simulink model "car_model2"  (R2023a)
settings: Solver=ode14x  StartTime=0.0  StopTime=40  FixedStep=0.001  RelTol=1e-3  EnableMultiTasking=on
undefined symbols (not defined in the file or in its folder): DiscIntNeverNeededParam, magnitude
settings Model: Creator=Sıla The Magnificent  LastModifiedBy=Sıla The Magnificent

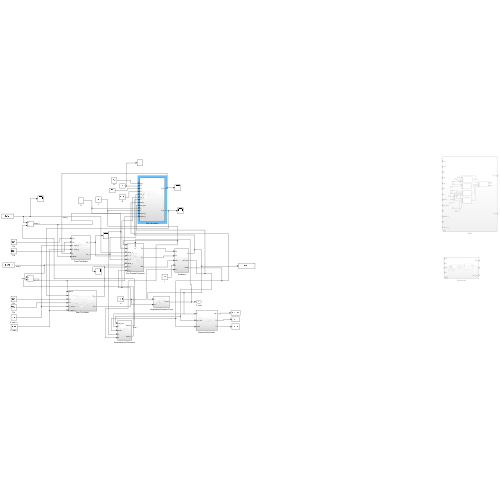
[thumbnail: Simulink's stored preview of the top-level diagram]
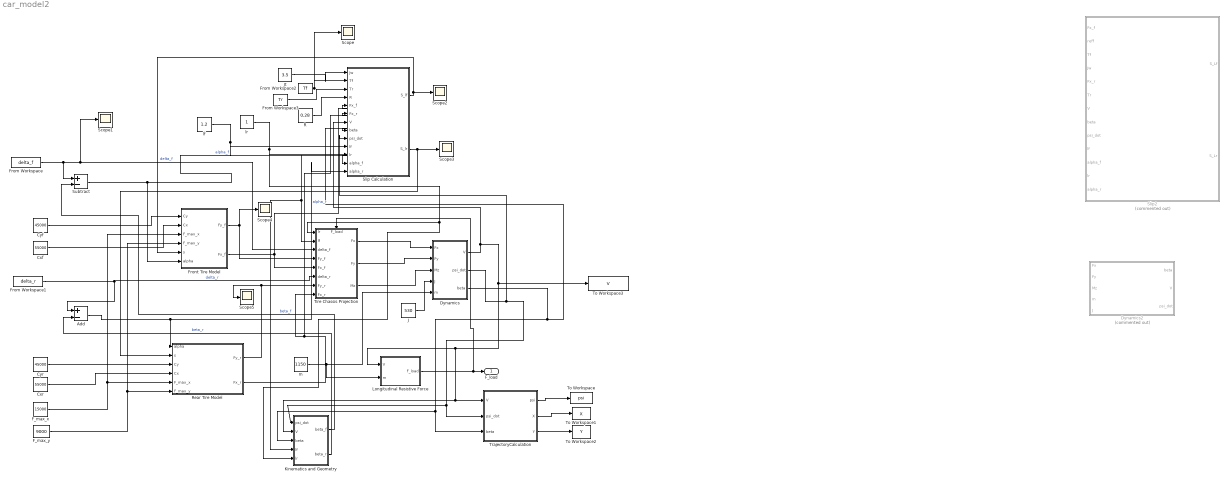
== system car_model2 ==
  Add : Sum  Inputs=+-
  Cxf : Constant  Value=55000
  Cxr : Constant  Value=55000
  Cyf : Constant  Value=45000
  Cyr : Constant  Value=45000
  Dynamics : Subsystem
  Dynamics2 : Subsystem  Commented=on
  F_max_x : Constant  Value=15000
  F_max_y : Constant  Value=9000
  From Workspace : FromWorkspace  VariableName=delta_f  OutputAfterFinalValue=Holding final value
  From Workspace1 : FromWorkspace  VariableName=delta_r  OutputAfterFinalValue=Holding final value
  From Workspace2 : FromWorkspace  VariableName=Tf  OutputAfterFinalValue=Holding final value
  From Workspace3 : FromWorkspace  VariableName=Tr  OutputAfterFinalValue=Holding final value
  Front Tire Model : Subsystem
  J : Constant  Value=530
  Jt : Constant  Value=3.5
  Kinematics and Geometry : Subsystem
  Longitudinal Resistive Force : Subsystem
  R : Constant  Value=0.28
  Rear Tire Model : Subsystem
  Scope{,1..5} (6 alike) : Scope
  Slip Calculation : Subsystem
  Slip2 : Subsystem  Commented=on
  Subtract : Sum  Inputs=+-
  Tire Chassis Projection : Subsystem
      settings: PortSchema="{\"entries\":[{\"content\":{\"sides\":[{\"content\":{\"connectorIds\":[\"In1\",\"In2\",\"In3\",\"In4\",\"In5\",\"In6\",\"In7\",\"In8\"]},\"type\":\"ConnectorPlacement.EquallySpacedRectSide\",\"uuid\":\"5673b256-c305-4d61-be24-85134e9539e3\"},{\"content\":{\"connectorIds\":[\"Out1\",\"Out2\",\"Out3\"],\"side\":\"RIGHT\"},\"type\":\"ConnectorPlacement.EquallySpacedRectSide\",\"uuid\":\"aa59e9e0-ca8f-48e9-aa74-948ec9a94037\"},{\"content\":{\"connectorIds\":[\"In9\"],\"side\":\"TOP\"},\"type\":\"ConnectorPlacement.EquallySpacedRectSide\",\"uuid\":\"62ad5797-b838-4702-bee2-dc097808f1bc\"}]},\"type\":\"ConnectorPlacement.EquallySpacedConnector\",\"uuid\":\"bd61d71e-e54e-45a1-97e3-844ee06cfb7b\"}],\"packageUris\":[\"http://schema.mathworks.com/mf0/Connector/R2020b\"],\"version\":\"1.0\"}"
  To Workspace : ToWorkspace  VariableName=psi  SaveFormat=Structure With Time  SampleTime=-1
  To Workspace1 : ToWorkspace  VariableName=X  SaveFormat=Structure With Time  SampleTime=-1
  To Workspace2 : ToWorkspace  VariableName=Y  SaveFormat=Structure With Time  SampleTime=-1
  To Workspace3 : ToWorkspace  VariableName=V  SaveFormat=Structure With Time  SampleTime=-1
  TrajectoryCalculation : Subsystem
  lf : Constant  Value=1.2
  lr : Constant
  m : Constant  Value=1150
  F_load : Outport
  wires:
  Cyf/1 -> Front Tire Model/1(Cy)
  Cxr/1 -> Rear Tire Model/4(Cx)
  Add/1 -> Rear Tire Model/1(alpha), Slip Calculation/13(alpha_r)  "alpha_r"
  Subtract/1 -> Slip Calculation/12(alpha_f), Front Tire Model/6(alpha)  "alpha_f"
  F_max_x/1 -> Front Tire Model/3(F_max_x), Rear Tire Model/5(F_max_x)
  F_max_y/1 -> Front Tire Model/4(F_max_y), Rear Tire Model/6(F_max_y)
  m/1 -> Dynamics/5(m), Longitudinal Resistive Force/2(m)
  Longitudinal Resistive Force/1(F_load) -> F_load/1, Tire Chassis Projection/9(F_load)
  lf/1 -> Kinematics and Geometry/4(lf), Tire Chassis Projection/2(lf), Slip Calculation/10(lf)
  lr/1 -> Slip Calculation/11(lr), Tire Chassis Projection/1(lr), Kinematics and Geometry/5(lr)
  Kinematics and Geometry/2(beta_r) -> Add/2  "beta_r"
  TrajectoryCalculation/3(Y) -> To Workspace2/1
  TrajectoryCalculation/1(psi) -> To Workspace/1
  From Workspace/1 -> Scope1/1, Tire Chassis Projection/3(delta_f), Subtract/1  "delta_f"
  Cxf/1 -> Front Tire Model/2(Cx)
  Cyr/1 -> Rear Tire Model/3(Cy)
  TrajectoryCalculation/2(X) -> To Workspace1/1
  Front Tire Model/2(Fx_f) -> Tire Chassis Projection/5(Fx_f), Slip Calculation/5(Fx_f)
  Front Tire Model/1(Fy_f) -> Scope4/1, Tire Chassis Projection/4(Fy_f)
  Rear Tire Model/1(Fy_r) -> Scope5/1, Tire Chassis Projection/7(Fy_r)
  Rear Tire Model/2(Fx_r) -> Tire Chassis Projection/8(Fx_r), Slip Calculation/6(Fx_r)
  Kinematics and Geometry/1(beta_f) -> Subtract/2  "beta_f"
  From Workspace1/1 -> Tire Chassis Projection/6(delta_r), Add/1  "delta_r"
  J/1 -> Dynamics/4(J)
  Dynamics/1(V) -> To Workspace3/1, TrajectoryCalculation/1(V), Kinematics and Geometry/2(V), Longitudinal Resistive Force/1(V), Slip Calculation/7(V)
  Tire Chassis Projection/1(Fx) -> Dynamics/1(Fx)
  Tire Chassis Projection/2(Fy) -> Dynamics/2(Fy)
  Tire Chassis Projection/3(Mz) -> Dynamics/3(Mz)
  Dynamics/2(psi_dot) -> TrajectoryCalculation/2(psi_dot), Kinematics and Geometry/1(psi_dot), Slip Calculation/9(psi_dot)
  Dynamics/3(beta) -> Slip Calculation/8(beta), TrajectoryCalculation/3(beta), Kinematics and Geometry/3(beta)
  Jt/1 -> Slip Calculation/1(Jw)
  From Workspace2/1 -> Scope/1, Slip Calculation/2(Tf)
  From Workspace3/1 -> Slip Calculation/3(Tr)
  R/1 -> Slip Calculation/4(R)
  Slip Calculation/2(S_lr) -> Scope3/1, Rear Tire Model/2(s)
  Slip Calculation/1(S_lf) -> Scope2/1, Front Tire Model/5(s)

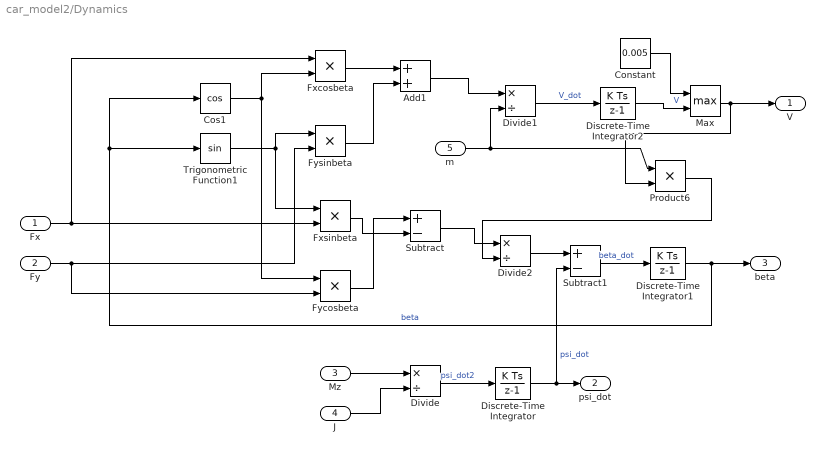
== system car_model2/Dynamics ==
  Fx : Inport
  Fy : Inport  Port=2
  Mz : Inport  Port=3
  J : Inport  Port=4
  m : Inport  Port=5
  Add1 : Sum
  Constant : Constant  Value=0.005
  Cos1 : Trigonometry  Operator=cos
  Discrete-Time Integrator : DiscreteIntegrator  SampleTime=-1  ICPrevOutput=DiscIntNeverNeededParam  ICPrevScaledInput=DiscIntNeverNeededParam
  Discrete-Time Integrator1 : DiscreteIntegrator  SampleTime=-1  ICPrevOutput=DiscIntNeverNeededParam  ICPrevScaledInput=DiscIntNeverNeededParam
  Discrete-Time Integrator2 : DiscreteIntegrator  SampleTime=-1  ICPrevOutput=DiscIntNeverNeededParam  ICPrevScaledInput=DiscIntNeverNeededParam
  Divide : Product  Inputs=*/
  Divide1 : Product  Inputs=*/
  Divide2 : Product  Inputs=*/
  Fxcosbeta : Product
  Fxsinbeta : Product
  Fycosbeta : Product
  Fysinbeta : Product
  Max : MinMax  Function=max  Inputs=2
  Product6 : Product
  Subtract : Sum  Inputs=+-
  Subtract1 : Sum  Inputs=+-
  Trigonometric Function1 : Trigonometry
  V : Outport
  psi_dot : Outport  Port=2
  beta : Outport  Port=3
  wires:
  m/1 -> Product6/1, Divide1/2
  Fy/1 -> Fycosbeta/2, Fysinbeta/2
  Discrete-Time Integrator1/1 -> beta/1, Trigonometric Function1/1, Cos1/1  "beta"
  Subtract/1 -> Divide2/1
  Trigonometric Function1/1 -> Fysinbeta/1, Fxsinbeta/1
  Fxsinbeta/1 -> Subtract/2
  Product6/1 -> Divide2/2
  Mz/1 -> Divide/1
  Fx/1 -> Fxsinbeta/2, Fxcosbeta/1
  Subtract1/1 -> Discrete-Time Integrator1/1  "beta_dot"
  Divide1/1 -> Discrete-Time Integrator2/1  "V_dot"
  Add1/1 -> Divide1/1
  Cos1/1 -> Fxcosbeta/2, Fycosbeta/1
  Divide/1 -> Discrete-Time Integrator/1  "psi_dot2"
  J/1 -> Divide/2
  Divide2/1 -> Subtract1/1
  Fycosbeta/1 -> Subtract/1
  Fysinbeta/1 -> Add1/2
  Fxcosbeta/1 -> Add1/1
  Discrete-Time Integrator/1 -> Subtract1/2, psi_dot/1  "psi_dot"
  Max/1 -> V/1, Product6/2
  Discrete-Time Integrator2/1 -> Max/2  "V"
  Constant/1 -> Max/1

== system car_model2/Dynamics2 ==
  Fx : Inport
  Fy : Inport  Port=2
  Mz : Inport  Port=3
  m : Inport  Port=4
  J : Inport  Port=5
  Discrete-Time Integrator : DiscreteIntegrator  SampleTime=-1  ICPrevOutput=DiscIntNeverNeededParam  ICPrevScaledInput=DiscIntNeverNeededParam
  Discrete-Time Integrator1 : DiscreteIntegrator  SampleTime=-1  ICPrevOutput=DiscIntNeverNeededParam  ICPrevScaledInput=DiscIntNeverNeededParam
  Discrete-Time Integrator2 : DiscreteIntegrator  SampleTime=-1  ICPrevOutput=DiscIntNeverNeededParam  ICPrevScaledInput=DiscIntNeverNeededParam
  IC : InitialCondition  Value=0
  first stage : MATLAB Function  TreatAsAtomicUnit=on
  second stage : MATLAB Function  TreatAsAtomicUnit=on
  beta : Outport
  V : Outport  Port=2
  psi_dot : Outport  Port=3
  wires:
  Fx/1 -> first stage/1(Fx)
  Fy/1 -> first stage/2(Fy)
  Mz/1 -> first stage/3(Mz)
  first stage/2(V_dot) -> Discrete-Time Integrator/1
  first stage/3(psi_double_dot) -> Discrete-Time Integrator1/1
  first stage/1(V_times_psidot_plus_betadot) -> second stage/1(V_times_psidot_plus_betadot)
  Discrete-Time Integrator/1 -> second stage/2(V), V/1
  Discrete-Time Integrator1/1 -> psi_dot/1, second stage/3(psi_dot)
  second stage/1(beta_dot) -> Discrete-Time Integrator2/1
  Discrete-Time Integrator2/1 -> IC/1, beta/1
  m/1 -> first stage/5(m)
  J/1 -> first stage/6(J)
  IC/1 -> first stage/4(beta)

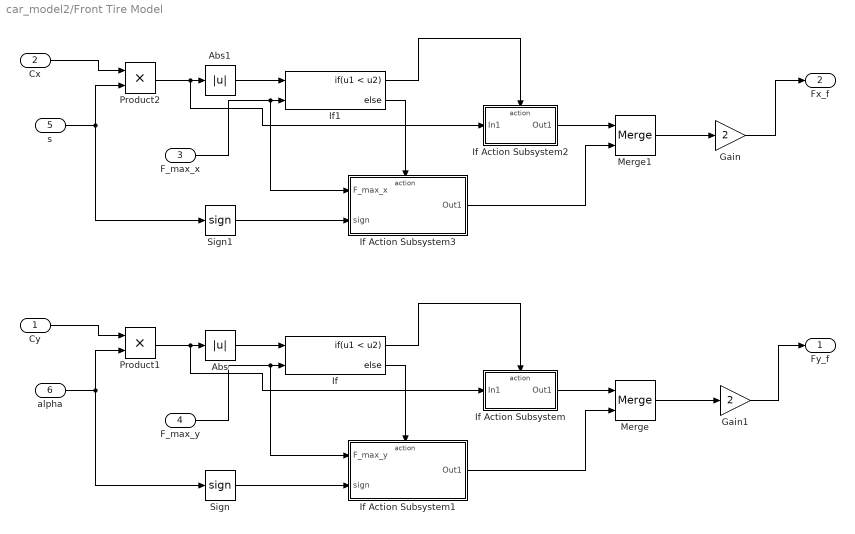
== system car_model2/Front Tire Model ==
  Cy : Inport
  Cx : Inport  Port=2
  F_max_x : Inport  Port=3
  F_max_y : Inport  Port=4
  s : Inport  Port=5
  alpha : Inport  Port=6
  Abs : Abs  SaturateOnIntegerOverflow=off
  Abs1 : Abs  SaturateOnIntegerOverflow=off
  Gain : Gain  Gain=2
  Gain1 : Gain  Gain=2
  If : If  NumInputs=2  IfExpression=u1 < u2
  If Action Subsystem : Subsystem  TreatAsAtomicUnit=on
  If Action Subsystem1 : Subsystem  TreatAsAtomicUnit=on
  If Action Subsystem2 : Subsystem  TreatAsAtomicUnit=on
  If Action Subsystem3 : Subsystem  TreatAsAtomicUnit=on
  If1 : If  NumInputs=2  IfExpression=u1 < u2
  Merge : Merge
  Merge1 : Merge
  Product1 : Product
  Product2 : Product
  Sign : Signum
  Sign1 : Signum
  Fy_f : Outport
  Fx_f : Outport  Port=2
  wires:
  F_max_x/1 -> If Action Subsystem3/1(F_max_x), If1/2
  If1/1 -> If Action Subsystem2/Action
  s/1 -> Sign1/1, Product2/2
  If Action Subsystem3/1(Out1) -> Merge1/2
  alpha/1 -> Sign/1, Product1/2
  Abs1/1 -> If1/1
  Sign/1 -> If Action Subsystem1/2(sign)
  Product2/1 -> If Action Subsystem2/1(In1), Abs1/1
  If Action Subsystem2/1(Out1) -> Merge1/1
  If/2 -> If Action Subsystem1/Action
  Cx/1 -> Product2/1
  Cy/1 -> Product1/1
  If1/2 -> If Action Subsystem3/Action
  Product1/1 -> If Action Subsystem/1(In1), Abs/1
  If Action Subsystem1/1(Out1) -> Merge/2
  Sign1/1 -> If Action Subsystem3/2(sign)
  If Action Subsystem/1(Out1) -> Merge/1
  F_max_y/1 -> If Action Subsystem1/1(F_max_y), If/2
  If/1 -> If Action Subsystem/Action
  Abs/1 -> If/1
  Merge1/1 -> Gain/1
  Gain/1 -> Fx_f/1
  Merge/1 -> Gain1/1
  Gain1/1 -> Fy_f/1

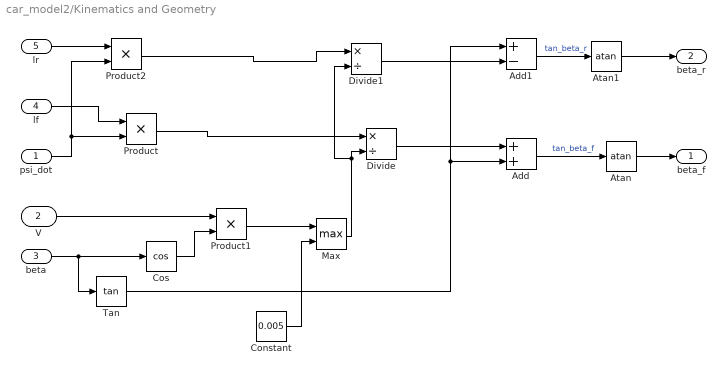
== system car_model2/Kinematics and Geometry ==
  psi_dot : Inport
  V : Inport  Port=2
  beta : Inport  Port=3
  lf : Inport  Port=4
  lr : Inport  Port=5
  Add : Sum
  Add1 : Sum  Inputs=+-
  Atan : Trigonometry  Operator=atan
  Atan1 : Trigonometry  Operator=atan
  Constant : Constant  Value=0.005
  Cos : Trigonometry  Operator=cos
  Divide : Product  Inputs=*/
  Divide1 : Product  Inputs=*/
  Max : MinMax  Function=max  Inputs=2
  Product : Product
  Product1 : Product
  Product2 : Product
  Tan : Trigonometry  Operator=tan
  beta_f : Outport
  beta_r : Outport  Port=2
  wires:
  lf/1 -> Product/1
  psi_dot/1 -> Product2/2, Product/2
  Product/1 -> Divide/1
  beta/1 -> Tan/1, Cos/1
  Cos/1 -> Product1/2
  Tan/1 -> Add1/1, Add/2
  Divide/1 -> Add/1
  Add/1 -> Atan/1  "tan_beta_f"
  Atan/1 -> beta_f/1
  lr/1 -> Product2/1
  Product2/1 -> Divide1/1
  Divide1/1 -> Add1/2
  Add1/1 -> Atan1/1  "tan_beta_r"
  Atan1/1 -> beta_r/1
  Constant/1 -> Max/2
  V/1 -> Product1/1
  Product1/1 -> Max/1
  Max/1 -> Divide1/2, Divide/2

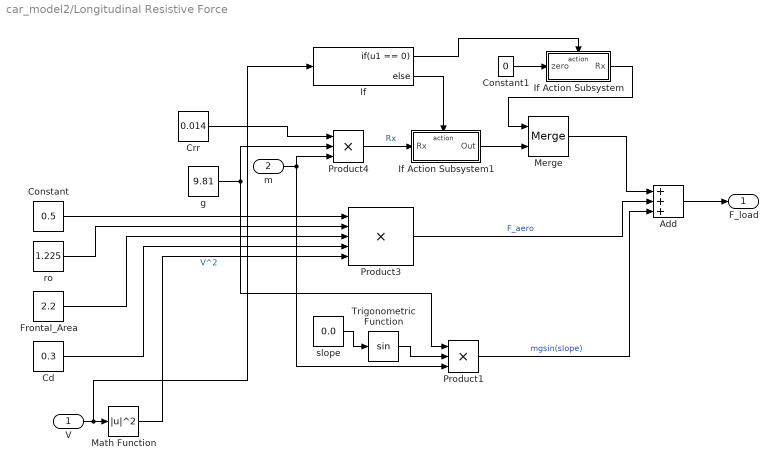
== system car_model2/Longitudinal Resistive Force ==
  V : Inport
  m : Inport  Port=2
  Add : Sum  Inputs=+++
  Cd : Constant  Value=0.3
  Constant : Constant  Value=0.5
  Constant1 : Constant  Value=0
  Crr : Constant  Value=0.014
  Frontal_Area : Constant  Value=2.2
  If : If  IfExpression=u1 == 0
  If Action Subsystem : Subsystem  TreatAsAtomicUnit=on
  If Action Subsystem1 : Subsystem  TreatAsAtomicUnit=on
  Math Function : Math  Operator=magnitude^2
  Merge : Merge
  Product1 : Product  Inputs=3
  Product3 : Product  Inputs=5
  Product4 : Product  Inputs=3
  Trigonometric Function : Trigonometry
  g : Constant  Value=9.81
  ro : Constant  Value=1.225
  slope : Constant  Value=0.0
  F_load : Outport
  wires:
  Frontal_Area/1 -> Product3/3
  Product4/1 -> If Action Subsystem1/1(Rx)  "Rx"
  Cd/1 -> Product3/4
  g/1 -> Product4/2, Product1/1
  Add/1 -> F_load/1
  Trigonometric Function/1 -> Product1/2
  m/1 -> Product1/3, Product4/3
  slope/1 -> Trigonometric Function/1
  Constant/1 -> Product3/1
  Product3/1 -> Add/2  "F_aero"
  ro/1 -> Product3/2
  Math Function/1 -> Product3/5  "V^2"
  Crr/1 -> Product4/1
  Product1/1 -> Add/3  "mgsin(slope)"
  V/1 -> If/1, Math Function/1
  If/1 -> If Action Subsystem/Action
  If/2 -> If Action Subsystem1/Action
  If Action Subsystem/1(Rx) -> Merge/1
  If Action Subsystem1/1(Out) -> Merge/2
  Merge/1 -> Add/1
  Constant1/1 -> If Action Subsystem/1(zero)

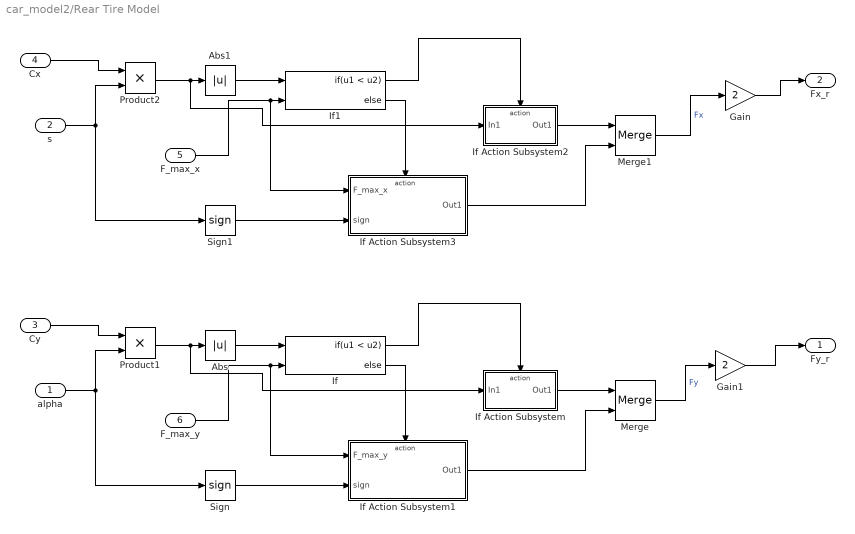
== system car_model2/Rear Tire Model ==
  alpha : Inport
  s : Inport  Port=2
  Cy : Inport  Port=3
  Cx : Inport  Port=4
  F_max_x : Inport  Port=5
  F_max_y : Inport  Port=6
  Abs : Abs  SaturateOnIntegerOverflow=off
  Abs1 : Abs  SaturateOnIntegerOverflow=off
  Gain : Gain  Gain=2
  Gain1 : Gain  Gain=2
  If : If  NumInputs=2  IfExpression=u1 < u2
  If Action Subsystem : Subsystem  TreatAsAtomicUnit=on
  If Action Subsystem1 : Subsystem  TreatAsAtomicUnit=on
  If Action Subsystem2 : Subsystem  TreatAsAtomicUnit=on
  If Action Subsystem3 : Subsystem  TreatAsAtomicUnit=on
  If1 : If  NumInputs=2  IfExpression=u1 < u2
  Merge : Merge
  Merge1 : Merge
  Product1 : Product
  Product2 : Product
  Sign : Signum
  Sign1 : Signum
  Fy_r : Outport
  Fx_r : Outport  Port=2
  wires:
  Sign1/1 -> If Action Subsystem3/2(sign)
  s/1 -> Sign1/1, Product2/2
  If/1 -> If Action Subsystem/Action
  If1/1 -> If Action Subsystem2/Action
  F_max_x/1 -> If Action Subsystem3/1(F_max_x), If1/2
  If Action Subsystem3/1(Out1) -> Merge1/2
  Sign/1 -> If Action Subsystem1/2(sign)
  If Action Subsystem2/1(Out1) -> Merge1/1
  F_max_y/1 -> If Action Subsystem1/1(F_max_y), If/2
  Abs1/1 -> If1/1
  alpha/1 -> Sign/1, Product1/2
  If Action Subsystem1/1(Out1) -> Merge/2
  If/2 -> If Action Subsystem1/Action
  Product2/1 -> If Action Subsystem2/1(In1), Abs1/1
  If1/2 -> If Action Subsystem3/Action
  Cx/1 -> Product2/1
  Product1/1 -> If Action Subsystem/1(In1), Abs/1
  If Action Subsystem/1(Out1) -> Merge/1
  Cy/1 -> Product1/1
  Abs/1 -> If/1
  Merge1/1 -> Gain/1  "Fx"
  Gain/1 -> Fx_r/1
  Merge/1 -> Gain1/1  "Fy"
  Gain1/1 -> Fy_r/1

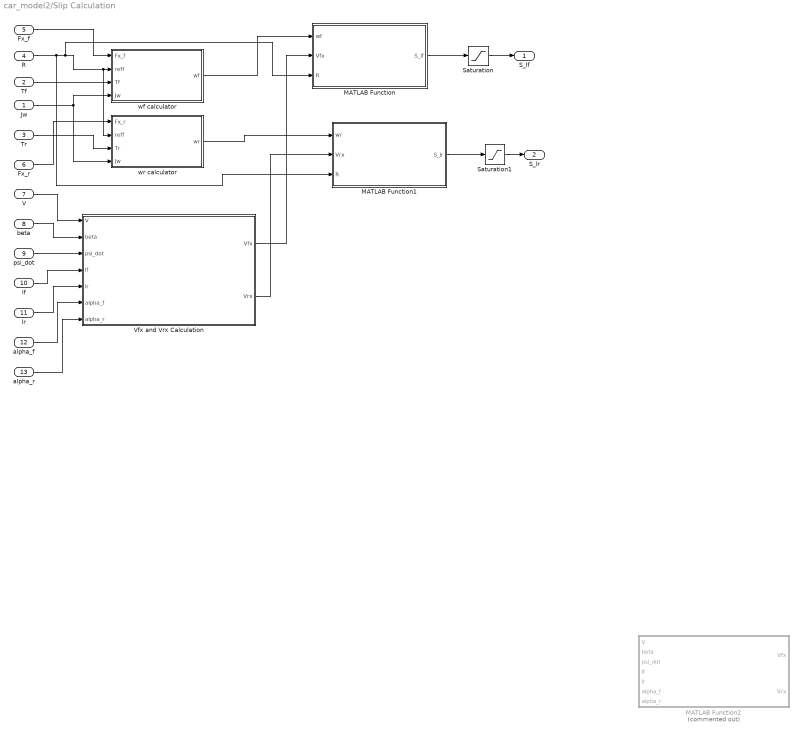
== system car_model2/Slip Calculation ==
  Jw : Inport
  Tf : Inport  Port=2
  Tr : Inport  Port=3
  R : Inport  Port=4
  Fx_f : Inport  Port=5
  Fx_r : Inport  Port=6
  V : Inport  Port=7
  beta : Inport  Port=8
  psi_dot : Inport  Port=9
  lf : Inport  Port=10
  lr : Inport  Port=11
  alpha_f : Inport  Port=12
  alpha_r : Inport  Port=13
  MATLAB Function : MATLAB Function  TreatAsAtomicUnit=on
  MATLAB Function1 : MATLAB Function  TreatAsAtomicUnit=on
  MATLAB Function2 : MATLAB Function  Commented=on  TreatAsAtomicUnit=on
  Saturation : Saturate  UpperLimit=1  LowerLimit=-1
  Saturation1 : Saturate  UpperLimit=1  LowerLimit=-1
  Vfx and Vrx Calculation : Subsystem
  wf calculator : Subsystem
  wr calculator : Subsystem
  S_lf : Outport
  S_lr : Outport  Port=2
  wires:
  Jw/1 -> wr calculator/4(Jw), wf calculator/4(Jw)
  Tr/1 -> wr calculator/3(Tr)
  Tf/1 -> wf calculator/3(Tf)
  Fx_f/1 -> wf calculator/1(Fx_f)
  Fx_r/1 -> wr calculator/1(Fx_r)
  V/1 -> Vfx and Vrx Calculation/1(V)
  beta/1 -> Vfx and Vrx Calculation/2(beta)
  psi_dot/1 -> Vfx and Vrx Calculation/3(psi_dot)
  lf/1 -> Vfx and Vrx Calculation/4(lf)
  lr/1 -> Vfx and Vrx Calculation/5(lr)
  alpha_f/1 -> Vfx and Vrx Calculation/6(alpha_f)
  alpha_r/1 -> Vfx and Vrx Calculation/7(alpha_r)
  R/1 -> MATLAB Function1/3(R), MATLAB Function/3(R), wr calculator/2(reff), wf calculator/2(reff)
  wf calculator/1(wf) -> MATLAB Function/1(wf)
  Vfx and Vrx Calculation/1(Vfx) -> MATLAB Function/2(Vfx)
  wr calculator/1(wr) -> MATLAB Function1/1(wr)
  Vfx and Vrx Calculation/2(Vrx) -> MATLAB Function1/2(Vrx)
  MATLAB Function1/1(S_lr) -> Saturation1/1
  MATLAB Function/1(S_lf) -> Saturation/1
  Saturation/1 -> S_lf/1
  Saturation1/1 -> S_lr/1

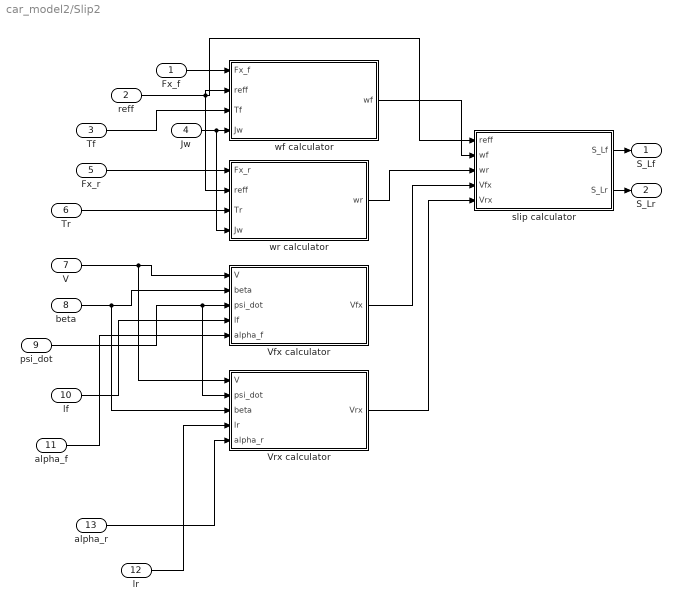
== system car_model2/Slip2 ==
  Fx_f : Inport
  reff : Inport  Port=2
  Tf : Inport  Port=3
  Jw : Inport  Port=4
  Fx_r : Inport  Port=5
  Tr : Inport  Port=6
  V : Inport  Port=7
  beta : Inport  Port=8
  psi_dot : Inport  Port=9
  lf : Inport  Port=10
  alpha_f : Inport  Port=11
  lr : Inport  Port=12
  alpha_r : Inport  Port=13
  Vfx calculator : Subsystem
  Vrx calculator : Subsystem
  slip calculator : Subsystem
  wf calculator : Subsystem
  wr calculator : Subsystem
  S_Lf : Outport
  S_Lr : Outport  Port=2
  wires:
  V/1 -> Vrx calculator/1(V), Vfx calculator/1(V)
  reff/1 -> slip calculator/1(reff), wr calculator/2(reff), wf calculator/2(reff)
  slip calculator/1(S_Lf) -> S_Lf/1
  wr calculator/1(wr) -> slip calculator/3(wr)
  Vfx calculator/1(Vfx) -> slip calculator/4(Vfx)
  Vrx calculator/1(Vrx) -> slip calculator/5(Vrx)
  psi_dot/1 -> Vrx calculator/2(psi_dot), Vfx calculator/3(psi_dot)
  lr/1 -> Vrx calculator/4(lr)
  wf calculator/1(wf) -> slip calculator/2(wf)
  Tr/1 -> wr calculator/3(Tr)
  Fx_f/1 -> wf calculator/1(Fx_f)
  alpha_r/1 -> Vrx calculator/5(alpha_r)
  Jw/1 -> wr calculator/4(Jw), wf calculator/4(Jw)
  Tf/1 -> wf calculator/3(Tf)
  alpha_f/1 -> Vfx calculator/5(alpha_f)
  beta/1 -> Vrx calculator/3(beta), Vfx calculator/2(beta)
  Fx_r/1 -> wr calculator/1(Fx_r)
  lf/1 -> Vfx calculator/4(lf)
  slip calculator/2(S_Lr) -> S_Lr/1

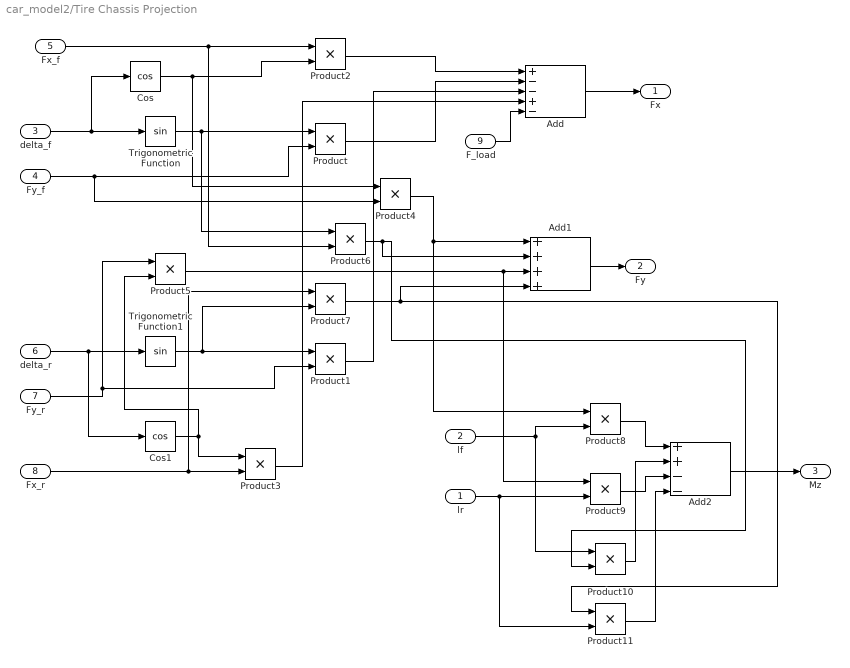
== system car_model2/Tire Chassis Projection ==
  lr : Inport
  lf : Inport  Port=2
  delta_f : Inport  Port=3
  Fy_f : Inport  Port=4
  Fx_f : Inport  Port=5
  delta_r : Inport  Port=6
  Fy_r : Inport  Port=7
  Fx_r : Inport  Port=8
  F_load : Inport  Port=9
  Add : Sum  Inputs=+--+-
  Add1 : Sum  Inputs=++++
  Add2 : Sum  Inputs=++--
  Cos : Trigonometry  Operator=cos
  Cos1 : Trigonometry  Operator=cos
  Product{,1..11} (12 alike) : Product
  Trigonometric Function : Trigonometry
  Trigonometric Function1 : Trigonometry
  Fx : Outport
  Fy : Outport  Port=2
  Mz : Outport  Port=3
  wires:
  delta_f/1 -> Cos/1, Trigonometric Function/1
  Trigonometric Function/1 -> Product/1, Product6/1
  Fy_f/1 -> Product4/2, Product/2
  delta_r/1 -> Cos1/1, Trigonometric Function1/1
  Trigonometric Function1/1 -> Product1/1, Product7/2
  Fy_r/1 -> Product5/1, Product1/2
  Cos/1 -> Product4/1, Product2/2
  Fx_f/1 -> Product6/2, Product2/1
  Cos1/1 -> Product5/2, Product3/1
  Fx_r/1 -> Product7/1, Product3/2
  Product2/1 -> Add/1
  Product/1 -> Add/2
  Product1/1 -> Add/3
  Product3/1 -> Add/4
  F_load/1 -> Add/5
  Add/1 -> Fx/1
  Product6/1 -> Product10/2, Add1/2
  Product4/1 -> Product8/1, Add1/1
  Product7/1 -> Product11/1, Add1/4
  Product5/1 -> Product9/1, Add1/3
  Add1/1 -> Fy/1
  lf/1 -> Product10/1, Product8/2
  lr/1 -> Product11/2, Product9/2
  Product8/1 -> Add2/1
  Product9/1 -> Add2/3
  Product10/1 -> Add2/2
  Product11/1 -> Add2/4
  Add2/1 -> Mz/1

== system car_model2/TrajectoryCalculation ==
  V : Inport
  psi_dot : Inport  Port=2
  beta : Inport  Port=3
  Add : Sum
  Cos : Trigonometry  Operator=cos
  Discrete-Time Integrator : DiscreteIntegrator  SampleTime=-1  ICPrevOutput=DiscIntNeverNeededParam  ICPrevScaledInput=DiscIntNeverNeededParam
  Discrete-Time Integrator1 : DiscreteIntegrator  SampleTime=-1  ICPrevOutput=DiscIntNeverNeededParam  ICPrevScaledInput=DiscIntNeverNeededParam
  Discrete-Time Integrator2 : DiscreteIntegrator  SampleTime=-1  ICPrevOutput=DiscIntNeverNeededParam  ICPrevScaledInput=DiscIntNeverNeededParam
  Product : Product
  Product1 : Product
  Trigonometric Function : Trigonometry
  psi : Outport
  X : Outport  Port=2
  Y : Outport  Port=3
  wires:
  Trigonometric Function/1 -> Product1/1
  Cos/1 -> Product/1
  Add/1 -> Cos/1, Trigonometric Function/1
  Discrete-Time Integrator1/1 -> X/1
  beta/1 -> Add/2
  Product1/1 -> Discrete-Time Integrator2/1
  V/1 -> Product/2, Product1/2
  Product/1 -> Discrete-Time Integrator1/1
  psi_dot/1 -> Discrete-Time Integrator/1
  Discrete-Time Integrator/1 -> Add/1, psi/1
  Discrete-Time Integrator2/1 -> Y/1

== system car_model2/Front Tire Model/If Action Subsystem ==
  In1 : Inport
  Action Port : ActionPort  ActionPortLabel=if(u1 < u2)
  Out1 : Outport
  wires:
  In1/1 -> Out1/1

== system car_model2/Front Tire Model/If Action Subsystem1 ==
  F_max_y : Inport
  sign : Inport  Port=2
  Action Port : ActionPort  ActionPortLabel=else
  Product : Product
  Out1 : Outport
  wires:
  Product/1 -> Out1/1
  F_max_y/1 -> Product/1
  sign/1 -> Product/2

== system car_model2/Front Tire Model/If Action Subsystem2 ==
  In1 : Inport
  Action Port : ActionPort  ActionPortLabel=if(u1 < u2)
  Out1 : Outport
  wires:
  In1/1 -> Out1/1

== system car_model2/Front Tire Model/If Action Subsystem3 ==
  F_max_x : Inport
  sign : Inport  Port=2
  Action Port : ActionPort  ActionPortLabel=else
  Product : Product
  Out1 : Outport
  wires:
  Product/1 -> Out1/1
  F_max_x/1 -> Product/1
  sign/1 -> Product/2

== system car_model2/Longitudinal Resistive Force/If Action Subsystem ==
  zero : Inport
  Action Port : ActionPort  ActionPortLabel=if(u1 == 0)
  Rx : Outport
  wires:
  zero/1 -> Rx/1

== system car_model2/Longitudinal Resistive Force/If Action Subsystem1 ==
  Rx : Inport
  Action Port : ActionPort  ActionPortLabel=else
  Out : Outport
  wires:
  Rx/1 -> Out/1

== system car_model2/Rear Tire Model/If Action Subsystem ==
  In1 : Inport
  Action Port : ActionPort  ActionPortLabel=if(u1 < u2)
  Out1 : Outport
  wires:
  In1/1 -> Out1/1

== system car_model2/Rear Tire Model/If Action Subsystem1 ==
  F_max_y : Inport
  sign : Inport  Port=2
  Action Port : ActionPort  ActionPortLabel=else
  Product : Product
  Out1 : Outport
  wires:
  Product/1 -> Out1/1
  F_max_y/1 -> Product/1
  sign/1 -> Product/2

== system car_model2/Rear Tire Model/If Action Subsystem2 ==
  In1 : Inport
  Action Port : ActionPort  ActionPortLabel=if(u1 < u2)
  Out1 : Outport
  wires:
  In1/1 -> Out1/1

== system car_model2/Rear Tire Model/If Action Subsystem3 ==
  F_max_x : Inport
  sign : Inport  Port=2
  Action Port : ActionPort  ActionPortLabel=else
  Product : Product
  Out1 : Outport
  wires:
  Product/1 -> Out1/1
  F_max_x/1 -> Product/1
  sign/1 -> Product/2

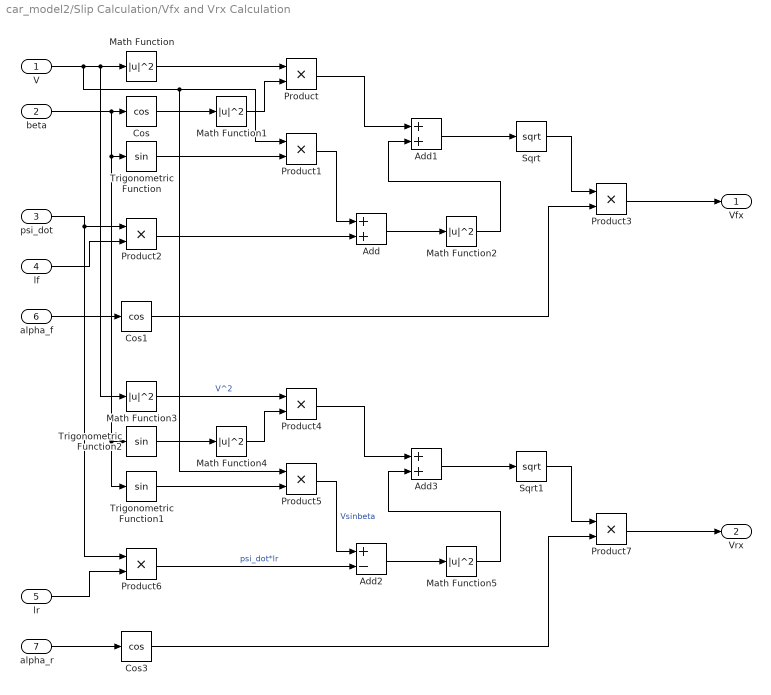
== system car_model2/Slip Calculation/Vfx and Vrx Calculation ==
  V : Inport
  beta : Inport  Port=2
  psi_dot : Inport  Port=3
  lf : Inport  Port=4
  lr : Inport  Port=5
  alpha_f : Inport  Port=6
  alpha_r : Inport  Port=7
  Add : Sum
  Add1 : Sum
  Add2 : Sum  Inputs=+-
  Add3 : Sum
  Cos : Trigonometry  Operator=cos
  Cos1 : Trigonometry  Operator=cos
  Cos3 : Trigonometry  Operator=cos
  Math Function{,1..5} (6 alike) : Math  Operator=magnitude^2
  Product{,1..7} (8 alike) : Product
  Sqrt : Sqrt
  Sqrt1 : Sqrt
  Trigonometric Function : Trigonometry
  Trigonometric Function1 : Trigonometry
  Trigonometric Function2 : Trigonometry
  Vfx : Outport
  Vrx : Outport  Port=2
  wires:
  V/1 -> Math Function/1, Math Function3/1, Product5/1, Product1/1
  Cos/1 -> Math Function1/1
  Math Function1/1 -> Product/2
  Math Function/1 -> Product/1
  Trigonometric Function/1 -> Product1/2
  lf/1 -> Product2/2
  Product2/1 -> Add/2
  Product1/1 -> Add/1
  Add/1 -> Math Function2/1
  Product/1 -> Add1/1
  Math Function2/1 -> Add1/2
  Add1/1 -> Sqrt/1
  alpha_f/1 -> Cos1/1
  Sqrt/1 -> Product3/1
  Cos1/1 -> Product3/2
  Product3/1 -> Vfx/1
  Product7/1 -> Vrx/1
  Math Function4/1 -> Product4/2
  alpha_r/1 -> Cos3/1
  Product5/1 -> Add2/1  "Vsinbeta"
  lr/1 -> Product6/2
  Math Function3/1 -> Product4/1  "V^2"
  Product4/1 -> Add3/1
  Sqrt1/1 -> Product7/1
  Trigonometric Function2/1 -> Math Function4/1
  Product6/1 -> Add2/2  "psi_dot*lr"
  Math Function5/1 -> Add3/2
  psi_dot/1 -> Product6/1, Product2/1
  Add3/1 -> Sqrt1/1
  Add2/1 -> Math Function5/1
  beta/1 -> Trigonometric Function2/1, Trigonometric Function1/1, Trigonometric Function/1, Cos/1
  Cos3/1 -> Product7/2
  Trigonometric Function1/1 -> Product5/2

== system car_model2/Slip Calculation/wf calculator ==
  Fx_f : Inport
  reff : Inport  Port=2
  Tf : Inport  Port=3
  Jw : Inport  Port=4
  Add : Sum  Inputs=+-
  Discrete-Time Integrator : DiscreteIntegrator  SampleTime=-1  ICPrevOutput=DiscIntNeverNeededParam  ICPrevScaledInput=DiscIntNeverNeededParam
  Divide : Product  Inputs=*/
  Product : Product
  wf : Outport
  wires:
  Fx_f/1 -> Product/1
  reff/1 -> Product/2
  Tf/1 -> Add/1
  Product/1 -> Add/2
  Add/1 -> Divide/1
  Jw/1 -> Divide/2
  Divide/1 -> Discrete-Time Integrator/1
  Discrete-Time Integrator/1 -> wf/1  "wf"

== system car_model2/Slip Calculation/wr calculator ==
  Fx_r : Inport
  reff : Inport  Port=2
  Tr : Inport  Port=3
  Jw : Inport  Port=4
  Add : Sum  Inputs=+-
  Discrete-Time Integrator : DiscreteIntegrator  SampleTime=-1  ICPrevOutput=DiscIntNeverNeededParam  ICPrevScaledInput=DiscIntNeverNeededParam
  Divide : Product  Inputs=*/
  Product : Product
  wr : Outport
  wires:
  Fx_r/1 -> Product/1
  reff/1 -> Product/2
  Tr/1 -> Add/1
  Product/1 -> Add/2
  Add/1 -> Divide/1
  Jw/1 -> Divide/2
  Divide/1 -> Discrete-Time Integrator/1
  Discrete-Time Integrator/1 -> wr/1

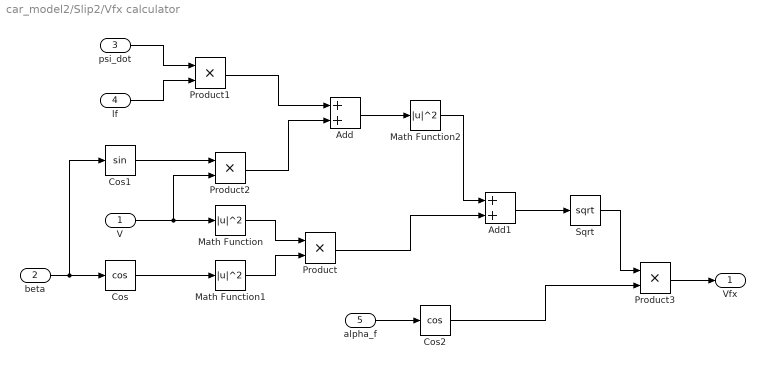
== system car_model2/Slip2/Vfx calculator ==
  V : Inport
  beta : Inport  Port=2
  psi_dot : Inport  Port=3
  lf : Inport  Port=4
  alpha_f : Inport  Port=5
  Add : Sum
  Add1 : Sum
  Cos : Trigonometry  Operator=cos
  Cos1 : Trigonometry
  Cos2 : Trigonometry  Operator=cos
  Math Function : Math  Operator=magnitude^2
  Math Function1 : Math  Operator=magnitude^2
  Math Function2 : Math  Operator=magnitude^2
  Product{,1..3} (4 alike) : Product
  Sqrt : Sqrt
  Vfx : Outport
  wires:
  beta/1 -> Cos1/1, Cos/1
  Cos/1 -> Math Function1/1
  V/1 -> Product2/2, Math Function/1
  Math Function/1 -> Product/1
  Math Function1/1 -> Product/2
  psi_dot/1 -> Product1/1
  lf/1 -> Product1/2
  Cos1/1 -> Product2/1
  Product1/1 -> Add/1
  Product2/1 -> Add/2
  Add/1 -> Math Function2/1
  Math Function2/1 -> Add1/1
  Product/1 -> Add1/2
  Add1/1 -> Sqrt/1
  alpha_f/1 -> Cos2/1
  Sqrt/1 -> Product3/1
  Cos2/1 -> Product3/2
  Product3/1 -> Vfx/1

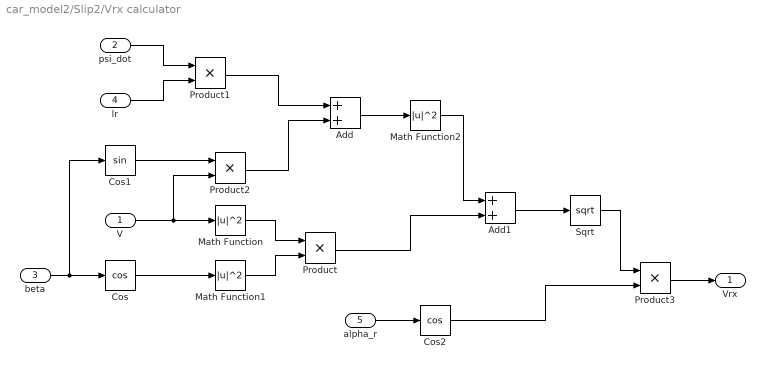
== system car_model2/Slip2/Vrx calculator ==
  V : Inport
  psi_dot : Inport  Port=2
  beta : Inport  Port=3
  lr : Inport  Port=4
  alpha_r : Inport  Port=5
  Add : Sum
  Add1 : Sum
  Cos : Trigonometry  Operator=cos
  Cos1 : Trigonometry
  Cos2 : Trigonometry  Operator=cos
  Math Function : Math  Operator=magnitude^2
  Math Function1 : Math  Operator=magnitude^2
  Math Function2 : Math  Operator=magnitude^2
  Product{,1..3} (4 alike) : Product
  Sqrt : Sqrt
  Vrx : Outport
  wires:
  beta/1 -> Cos1/1, Cos/1
  Cos/1 -> Math Function1/1
  V/1 -> Product2/2, Math Function/1
  Math Function/1 -> Product/1
  Math Function1/1 -> Product/2
  psi_dot/1 -> Product1/1
  lr/1 -> Product1/2
  Cos1/1 -> Product2/1
  Product1/1 -> Add/1
  Product2/1 -> Add/2
  Add/1 -> Math Function2/1
  Math Function2/1 -> Add1/1
  Product/1 -> Add1/2
  Add1/1 -> Sqrt/1
  alpha_r/1 -> Cos2/1
  Sqrt/1 -> Product3/1
  Cos2/1 -> Product3/2
  Product3/1 -> Vrx/1

== system car_model2/Slip2/slip calculator ==
  reff : Inport
  wf : Inport  Port=2
  wr : Inport  Port=3
  Vfx : Inport  Port=4
  Vrx : Inport  Port=5
  If : If  NumInputs=2  IfExpression=u1 > u2  ElseIfExpressions=u1 < u2
  If Action Subsystem : Subsystem  TreatAsAtomicUnit=on
  If Action Subsystem1 : Subsystem  TreatAsAtomicUnit=on
  If Action Subsystem2 : Subsystem  TreatAsAtomicUnit=on
  If Action Subsystem3 : Subsystem  TreatAsAtomicUnit=on
  If Action Subsystem4 : Subsystem  TreatAsAtomicUnit=on
  If Action Subsystem5 : Subsystem  TreatAsAtomicUnit=on
  If1 : If  NumInputs=2  IfExpression=u1 > u2  ElseIfExpressions=u1 < u2
  Merge : Merge  Inputs=3
  Merge1 : Merge  Inputs=3
  Product : Product
  Product1 : Product
  S_Lf : Outport
  S_Lr : Outport  Port=2
  wires:
  wf/1 -> Product/1
  Product/1 -> If/2, If Action Subsystem/1(wfR), If Action Subsystem1/1(wfR)
  Vfx/1 -> If Action Subsystem/2(Vfx), If/1, If Action Subsystem1/2(Vfx)
  If/1 -> If Action Subsystem/Action  "braking"
  Merge/1 -> S_Lf/1
  If Action Subsystem/1(slip) -> Merge/1
  If Action Subsystem1/1(slip) -> Merge/3
  Merge1/1 -> S_Lr/1
  If Action Subsystem3/1(slip) -> Merge1/3
  wr/1 -> Product1/1
  If Action Subsystem2/1(slip) -> Merge1/1
  Product1/1 -> If1/2, If Action Subsystem2/1(wrR), If Action Subsystem3/1(wrR)
  reff/1 -> Product/2, Product1/2
  If1/1 -> If Action Subsystem2/Action  "braking"
  Vrx/1 -> If Action Subsystem2/2(Vrx), If1/1, If Action Subsystem3/2(Vrx)
  If/2 -> If Action Subsystem1/Action  "accelerating"
  If/3 -> If Action Subsystem4/Action
  If Action Subsystem4/1(slip) -> Merge/2
  If1/2 -> If Action Subsystem3/Action  "accelerating"
  If1/3 -> If Action Subsystem5/Action
  If Action Subsystem5/1(slip) -> Merge1/2

== system car_model2/Slip2/wf calculator ==
  Fx_f : Inport
  reff : Inport  Port=2
  Tf : Inport  Port=3
  Jw : Inport  Port=4
  Add : Sum  Inputs=+-
  Divide : Product  Inputs=*/
  Integrator : Integrator
  Product : Product
  wf : Outport
  wires:
  Fx_f/1 -> Product/1
  reff/1 -> Product/2
  Tf/1 -> Add/1
  Product/1 -> Add/2
  Add/1 -> Divide/1
  Jw/1 -> Divide/2
  Divide/1 -> Integrator/1
  Integrator/1 -> wf/1  "wf"

== system car_model2/Slip2/wr calculator ==
  Fx_r : Inport
  reff : Inport  Port=2
  Tr : Inport  Port=3
  Jw : Inport  Port=4
  Add : Sum  Inputs=+-
  Divide : Product  Inputs=*/
  Integrator : Integrator
  Product : Product
  wr : Outport
  wires:
  Fx_r/1 -> Product/1
  reff/1 -> Product/2
  Tr/1 -> Add/1
  Product/1 -> Add/2
  Add/1 -> Divide/1
  Jw/1 -> Divide/2
  Integrator/1 -> wr/1  "wr"
  Divide/1 -> Integrator/1

== system car_model2/Slip2/slip calculator/If Action Subsystem ==
  wfR : Inport
  Vfx : Inport  Port=2
  Action Port : ActionPort  ActionPortLabel=if(u1 > u2)
  Add : Sum  Inputs=+-
  Constant : Constant  Value=0.005
  Divide : Product  Inputs=*/
  Max : MinMax  Function=max  Inputs=2
  slip : Outport
  wires:
  wfR/1 -> Add/1
  Add/1 -> Divide/1
  Divide/1 -> slip/1
  Max/1 -> Add/2, Divide/2
  Constant/1 -> Max/2
  Vfx/1 -> Max/1

== system car_model2/Slip2/slip calculator/If Action Subsystem1 ==
  wfR : Inport
  Vfx : Inport  Port=2
  Action Port : ActionPort  ActionPortLabel=elseif(u1 < u2)
  Add : Sum  Inputs=+-
  Constant : Constant  Value=0.005
  Divide : Product  Inputs=*/
  Max : MinMax  Function=max  Inputs=2
  slip : Outport
  wires:
  Vfx/1 -> Add/2
  Add/1 -> Divide/1
  Divide/1 -> slip/1
  Constant/1 -> Max/2
  wfR/1 -> Max/1
  Max/1 -> Divide/2, Add/1

== system car_model2/Slip2/slip calculator/If Action Subsystem2 ==
  wrR : Inport
  Vrx : Inport  Port=2
  Action Port : ActionPort  ActionPortLabel=if(u1 > u2)
  Add : Sum  Inputs=+-
  Constant : Constant  Value=0.005
  Divide : Product  Inputs=*/
  Max : MinMax  Function=max  Inputs=2
  slip : Outport
  wires:
  wrR/1 -> Add/1
  Add/1 -> Divide/1
  Divide/1 -> slip/1
  Constant/1 -> Max/2
  Vrx/1 -> Max/1
  Max/1 -> Divide/2, Add/2

== system car_model2/Slip2/slip calculator/If Action Subsystem3 ==
  wrR : Inport
  Vrx : Inport  Port=2
  Action Port : ActionPort  ActionPortLabel=elseif(u1 < u2)
  Add : Sum  Inputs=+-
  Constant : Constant  Value=0.005
  Divide : Product  Inputs=*/
  Max : MinMax  Function=max  Inputs=2
  slip : Outport
  wires:
  Vrx/1 -> Add/2
  Add/1 -> Divide/1
  Divide/1 -> slip/1
  Constant/1 -> Max/2
  wrR/1 -> Max/1
  Max/1 -> Divide/2, Add/1

== system car_model2/Slip2/slip calculator/If Action Subsystem4 ==
  Action Port : ActionPort  ActionPortLabel=else
  Constant : Constant  Value=0
  slip : Outport
  wires:
  Constant/1 -> slip/1

== system car_model2/Slip2/slip calculator/If Action Subsystem5 ==
  Action Port : ActionPort  ActionPortLabel=else
  Constant : Constant  Value=0
  slip : Outport
  wires:
  Constant/1 -> slip/1

== matlab function car_model2/Dynamics2/first stage ==
  data: Fx input; V_times_psidot_plus_betadot output; Fy input; Mz input; V_dot output; psi_double_dot output; beta input; m input; J input
function[V_times_psidot_plus_betadot, V_dot, psi_double_dot] = fcn(Fx, Fy, Mz, beta, m, J)

    % Rotation matrix components
    R11 = -sin(beta);
    R12 = cos(beta);
    R21 = cos(beta);
    R22 = sin(beta);

    % Compute components of the result vector
    first_eq = R11 * Fx + R12 * Fy;         % corresponds to m*V*(beta_dot + psi_dot)
    second_eq = R21 * Fx + R22 * Fy;        % corresponds to m * V_dot
    third_eq = Mz;                          % corresponds to J * psi_double_dot

    % Output variables
    V_times_psidot_plus_betadot = first_eq / m;
    V_dot = second_eq / m;
    psi_double_dot = third_eq / J;
end

== matlab function car_model2/Dynamics2/second stage ==
  data: V_times_psidot_plus_betadot input; beta_dot output; V input; psi_dot input
function beta_dot  = fcn(V_times_psidot_plus_betadot, V, psi_dot)

    % Avoid division by zero
    if V == 0
        beta_dot = 0;
        return;
    end

    % Compute beta_dot
    beta_dot = (V_times_psidot_plus_betadot - V * psi_dot) / V;
end

== matlab function car_model2/Slip Calculation/MATLAB Function ==
  data: wf input; S_lf output; Vfx input; R input
function S_lf = S_lf_Calculation(wf, Vfx, R)

Vw = wf * R;

% To avoid division by zero
epsilon = 1e-6;

if Vw < Vfx - epsilon  % Braking
    S_lf = (Vw - Vfx) / Vfx;
elseif Vw > Vfx + epsilon  % Acceleration
    S_lf = (Vw - Vfx) / Vw;
else  % No slip 
    S_lf = 0;
end
end

== matlab function car_model2/Slip Calculation/MATLAB Function1 ==
  data: wr input; S_lr output; Vrx input; R input
function S_lr = S_lr_Calculation(wr, Vrx, R)

Vw = wr * R;

% Avoid division by zero
epsilon = 1e-6;

if Vw < Vrx - epsilon  % Braking
    S_lr = (Vw - Vrx) / Vrx;
elseif Vw > Vrx + epsilon  % Acceleration
    S_lr = (Vw - Vrx) / Vw;
else  % No slip
    S_lr = 0;
end
end

== matlab function car_model2/Slip Calculation/MATLAB Function2 ==
  data: V input; Vfx output; beta input; psi_dot input; lf input; lr input; alpha_f input; alpha_r input; Vrx output
function [Vfx, Vrx] = compute_axial_wheel_velocities(V, beta, psi_dot, lf, lr, alpha_f, alpha_r)

% Front
term1_f = V^2 * cos(beta)^2;
term2_f = (V * sin(beta) + psi_dot * lf)^2;
Vfx = sqrt(term1_f + term2_f) * cos(alpha_f);

% Rear
term1_r = V^2 * sin(beta)^2;
term2_r = (V * sin(beta) - psi_dot * lr)^2;
Vrx = sqrt(term1_r + term2_r)* cos(alpha_r);

end
